simulink model "lab_2_MC"  (Simulink 7.3)
settings: Solver=ode3  StartTime=0.0  StopTime=100000.0  FixedStep=1  RelTol=1e-3
undefined symbols (not defined in the file or in its folder): DiscIntNeverNeededParam
settings Model: Creator=IEUser  LastModifiedBy=IEUser
settings OptimizationCC: BooleanDataType=off

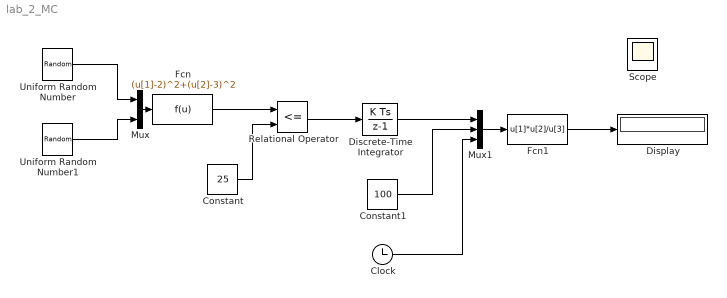
== system lab_2_MC ==
  Clock : Clock
      settings: Decimation=10
  Constant : Constant  Value=25  OutDataType=fixdt(1, 16)  OutScaling=2^0
  Constant1 : Constant  Value=100  OutDataType=fixdt(1, 16)  OutScaling=2^0
  Discrete-Time Integrator : DiscreteIntegrator  OutDataTypeMode=double  OutDataType=fixdt(1, 16)  OutScaling=2^0  OutDataTypeStr=double  ICPrevOutput=DiscIntNeverNeededParam  ICPrevScaledInput=DiscIntNeverNeededParam
  Display : Display
  Fcn : Fcn  Expr=(u[1]-2)^2+(u[2]-3)^2
  Fcn1 : Fcn  Expr=u[1]*u[2]/u[3]
  Mux : Mux  Inputs=2
  Mux1 : Mux  Inputs=3
  Relational Operator : RelationalOperator  Operator=<=  LogicOutDataTypeMode=boolean  LogicDataType=fixdt(0, 8)  OutDataTypeStr=boolean
  Scope : Scope
      settings: YMin=0  YMax=105
  Uniform Random Number : UniformRandomNumber  Minimum=-3  Maximum=7  SampleTime=0
  Uniform Random Number1 : UniformRandomNumber  Minimum=-2  Maximum=8  Seed=11  SampleTime=0
  wires:
  Uniform Random Number/1 -> Mux/1
  Uniform Random Number1/1 -> Mux/2
  Mux/1 -> Fcn/1
  Constant/1 -> Relational Operator/2
  Fcn/1 -> Relational Operator/1
  Relational Operator/1 -> Discrete-Time Integrator/1
  Discrete-Time Integrator/1 -> Mux1/1
  Constant1/1 -> Mux1/2
  Clock/1 -> Mux1/3
  Mux1/1 -> Fcn1/1
  Fcn1/1 -> Display/1
